simulink model "TFSimulink"  (R2016b)
settings: Solver=VariableStepAuto  StartTime=0.0  StopTime=100  RelTol=1e-3
undefined symbols (not defined in the file or in its folder): G
settings Model: Creator=Akash  LastModifiedBy=Akash

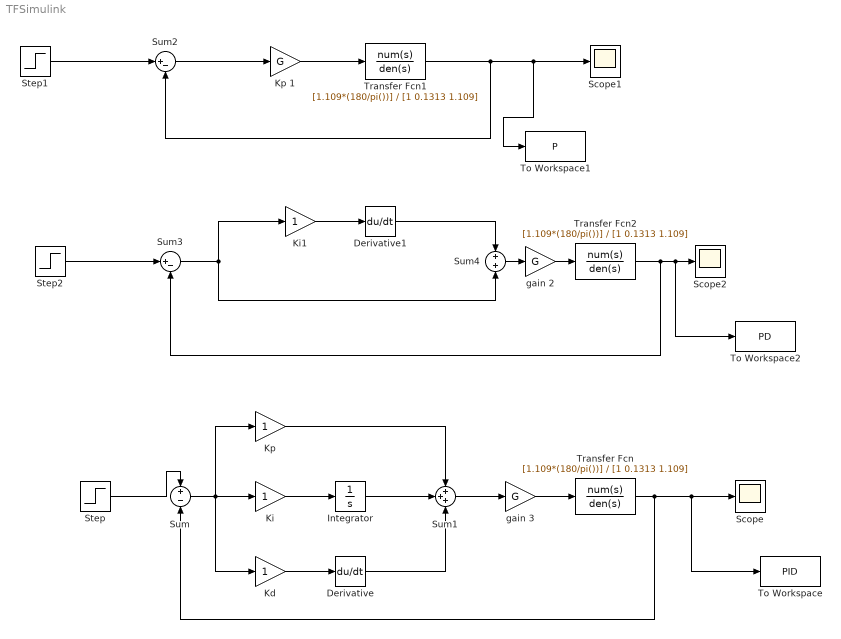
== system TFSimulink ==
  Derivative : Derivative
  Derivative1 : Derivative
  Integrator : Integrator
  "Kd " : Gain
  Ki : Gain
  Ki1 : Gain
  "Kp " : Gain
  Kp 1 : Gain  Gain=G
  Scope : Scope
  Scope1 : Scope
  Scope2 : Scope
  Step : Step  SampleTime=0
  Step1 : Step  SampleTime=0
  Step2 : Step  SampleTime=0
  Sum : Sum  Inputs=+-
  Sum1 : Sum  Inputs=+++
  Sum2 : Sum  Inputs=|+-
  Sum3 : Sum  Inputs=|+-
  Sum4 : Sum
  To Workspace : ToWorkspace  VariableName=PID  SaveFormat=Timeseries  SampleTime=-1
  To Workspace1 : ToWorkspace  VariableName=P  SaveFormat=Timeseries  SampleTime=-1
  To Workspace2 : ToWorkspace  VariableName=PD  SaveFormat=Timeseries  SampleTime=-1
  Transfer Fcn : TransferFcn  Numerator=[1.109*(180/pi())]  Denominator=[1 0.1313 1.109]
  Transfer Fcn1 : TransferFcn  Numerator=[1.109*(180/pi())]  Denominator=[1 0.1313 1.109]
  Transfer Fcn2 : TransferFcn  Numerator=[1.109*(180/pi())]  Denominator=[1 0.1313 1.109]
  gain 2 : Gain  Gain=G
  gain 3 : Gain  Gain=G
  wires:
  Transfer Fcn/1 -> To Workspace/1, Scope/1, Sum/2
  Step/1 -> Sum/1
  Sum/1 -> "Kp "/1, "Kd "/1, Ki/1
  Ki/1 -> Integrator/1
  Integrator/1 -> Sum1/2
  "Kd "/1 -> Derivative/1
  Derivative/1 -> Sum1/3
  Step1/1 -> Sum2/1
  Sum2/1 -> Kp 1/1
  Kp 1/1 -> Transfer Fcn1/1
  Transfer Fcn1/1 -> Sum2/2, To Workspace1/1, Scope1/1
  Step2/1 -> Sum3/1
  Sum3/1 -> Sum4/2, Ki1/1
  Ki1/1 -> Derivative1/1
  Transfer Fcn2/1 -> Sum3/2, To Workspace2/1, Scope2/1
  Sum4/1 -> gain 2/1
  gain 2/1 -> Transfer Fcn2/1
  Derivative1/1 -> Sum4/1
  "Kp "/1 -> Sum1/1
  Sum1/1 -> gain 3/1
  gain 3/1 -> Transfer Fcn/1
